simulink model "sensorfusion_omni_VxVyW"  (R2020b)
settings: Solver=ode1  StartTime=0.0  StopTime=100  FixedStep=0.01  RelTol=1e-3
settings Model: Creator=ONLY-GOD  LastModifiedBy=ONLY-GOD

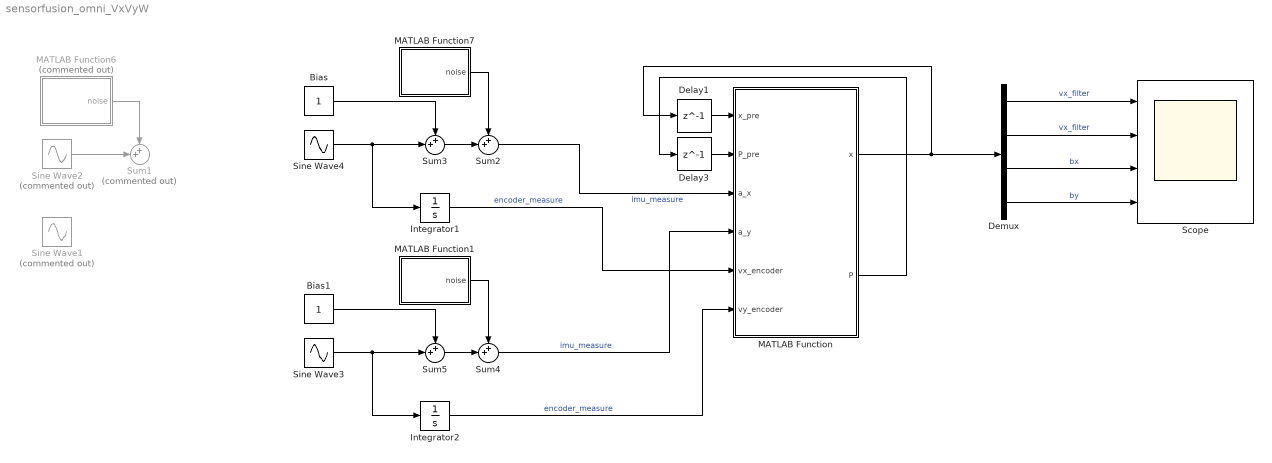
== system sensorfusion_omni_VxVyW ==
  Bias : Constant
  Bias1 : Constant
  Delay1 : Delay  DelayLength=1  InitialCondition=[0;0;0;0]
  Delay3 : Delay  DelayLength=1  InitialCondition=2*eye(4);
  Demux : Demux
  Integrator1 : Integrator
  Integrator2 : Integrator
  MATLAB Function : MATLAB Function  TreatAsAtomicUnit=on
  MATLAB Function1 : MATLAB Function  TreatAsAtomicUnit=on
  MATLAB Function6 : MATLAB Function  Commented=on  TreatAsAtomicUnit=on
  MATLAB Function7 : MATLAB Function  TreatAsAtomicUnit=on
  Scope : Scope  NumInputPorts=4
  Sine Wave1 : Sin  Commented=on  Amplitude=5  Frequency=0.1
  Sine Wave2 : Sin  Commented=on  Amplitude=5  Bias=1  Frequency=0.1
  Sine Wave3 : Sin  Amplitude=5  Frequency=0.1
  Sine Wave4 : Sin  Amplitude=5  Frequency=0.1
  Sum1 : Sum  Commented=on  Inputs=++|
  Sum{2..5} (4 alike) : Sum  Inputs=++|
  wires:
  Demux/4 -> Scope/4  "by"
  Demux/3 -> Scope/3  "bx"
  MATLAB Function/2(P) -> Delay3/1
  Sine Wave4/1 -> Sum3/2, Integrator1/1
  Demux/2 -> Scope/2  "vx_filter"
  Sum3/1 -> Sum2/2
  MATLAB Function6/1(noise) -> Sum1/1
  Delay3/1 -> MATLAB Function/2(P_pre)
  Demux/1 -> Scope/1  "vx_filter"
  Bias/1 -> Sum3/1
  MATLAB Function7/1(noise) -> Sum2/1
  Sine Wave2/1 -> Sum1/2
  MATLAB Function/1(x) -> Demux/1, Delay1/1
  Delay1/1 -> MATLAB Function/1(x_pre)
  MATLAB Function1/1(noise) -> Sum4/1
  Bias1/1 -> Sum5/1
  Sum5/1 -> Sum4/2
  Sine Wave3/1 -> Integrator2/1, Sum5/2
  Sum2/1 -> MATLAB Function/3(a_x)  "imu_measure"
  Integrator1/1 -> MATLAB Function/5(vx_encoder)  "encoder_measure"
  Sum4/1 -> MATLAB Function/4(a_y)  "imu_measure"
  Integrator2/1 -> MATLAB Function/6(vy_encoder)  "encoder_measure"

== matlab function sensorfusion_omni_VxVyW/MATLAB Function1 ==
  data: noise output
function noise = fnc()

noise = randn*0.1;

== matlab function sensorfusion_omni_VxVyW/MATLAB Function ==
  data: x_pre input; P_pre input; a_x input; a_y input; x output; vx_encoder input; P output; vy_encoder input
function [x,P] = kalman_filter(x_pre,P_pre,a_x,a_y,vx_encoder,vy_encoder)
% predefined
Ts = 0.01;
Q = 1e-1*diag([2 2 2 2]);
R = 1e-3*diag([1 1]);


% model prediction
A = [1 0 Ts 0;
     0 1 0 Ts;
     0 0 1  0;
     0 0 0  1];
B = [Ts 0;
     0 Ts;
     0  0;
     0  0];
C = [1 0 0 0;
     0 1 0 0];

u = [a_x;
     a_y];

x = A*x_pre + B*u;
P = A*P_pre*A' + Q;


%update
y = [vx_encoder;
     vy_encoder];
erry = y - C*x;
P_xz = P*C';
P_zz = C*P*C' + R;
x = x + (P_xz/P_zz)*erry;
P = P - (P_xz/P_zz)*P_xz';

== matlab function sensorfusion_omni_VxVyW/MATLAB Function6 ==
  data: noise output
function noise = fnc()

noise = randn*0.1;

== matlab function sensorfusion_omni_VxVyW/MATLAB Function7 ==
  data: noise output
function noise = fnc()

noise = randn*0.1;
